simulink model "v3_sim_pi"  (R2023b)
settings: Solver=VariableStepAuto  StartTime=0.0  StopTime=100  RelTol=1e-3
libraries: simulink x1
settings Model: Creator=kiraa  LastModifiedBy=kiraa

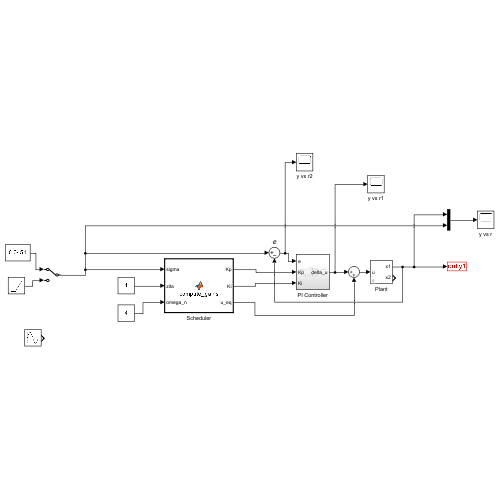
[thumbnail: Simulink's stored preview of the top-level diagram]
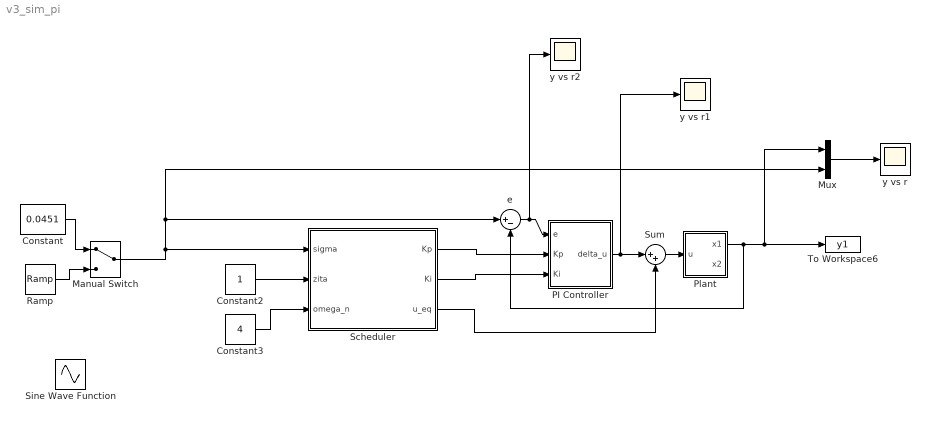
== system v3_sim_pi ==
  Constant : Constant  Value=0.0451
  Constant2 : Constant
  Constant3 : Constant  Value=4
  Manual Switch : ManualSwitch
  Mux : Mux  Inputs=2
  PI Controller : Subsystem
  Plant : Subsystem  mask{x1_0=0, x2_0=0}
      mask prompts: x1_0 "x1(0) [g/l]"; x2_0 "x2(0) [min^-1]"
  Ramp : simulink/Sources/Ramp  slope=0.00001  start=0  InitialOutput=0
  Scheduler : MATLAB Function  TreatAsAtomicUnit=on
  Sine Wave Function : Sin  Amplitude=0.001  Bias=0.0451  Frequency=0.1  SampleTime=0
  Sum : Sum  Inputs=|++
  To Workspace6 : ToWorkspace  VariableName=y1  SaveFormat=Timeseries  SampleTime=-1
  e : Sum  Inputs=|+-
  y vs r : Scope
  y vs r1 : Scope
  y vs r2 : Scope
  wires:
  Plant/1(x1) -> Mux/1, To Workspace6/1, e/2
  Mux/1 -> y vs r/1
  Constant/1 -> Manual Switch/1
  Manual Switch/1 -> Mux/2, e/1, Scheduler/1(sigma)
  Scheduler/1(Kp) -> PI Controller/2(Kp)
  Scheduler/2(Ki) -> PI Controller/3(Ki)
  Constant2/1 -> Scheduler/2(zita)
  Constant3/1 -> Scheduler/3(omega_n)
  Scheduler/3(u_eq) -> Sum/2
  PI Controller/1(delta_u) -> Sum/1, y vs r1/1
  e/1 -> y vs r2/1, PI Controller/1(e)
  Ramp/1 -> Manual Switch/2
  Sum/1 -> Plant/1(u)

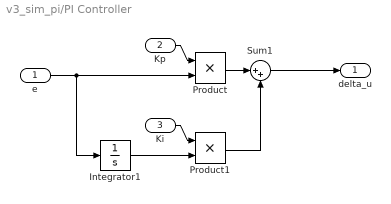
== system v3_sim_pi/PI Controller ==
  e : Inport
  Kp : Inport  Port=2
  Ki : Inport  Port=3
  Integrator1 : Integrator
  Product : Product
  Product1 : Product
  Sum1 : Sum  Inputs=|++
  delta_u : Outport
  wires:
  Product1/1 -> Sum1/2
  e/1 -> Product/2, Integrator1/1
  Integrator1/1 -> Product1/2
  Product/1 -> Sum1/1
  Ki/1 -> Product1/1
  Sum1/1 -> delta_u/1
  Kp/1 -> Product/1

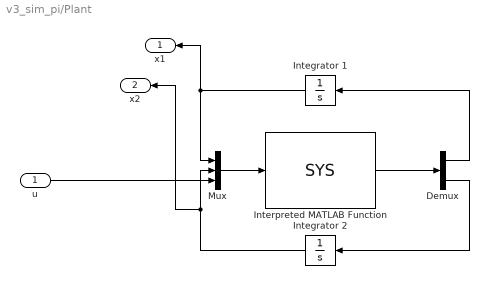
== system v3_sim_pi/Plant ==
  u : Inport
  Demux : Demux  Outputs=2
  Integrator 1 : Integrator  InitialCondition=x1_0
  Integrator 2 : Integrator  InitialCondition=x2_0
  Interpreted MATLAB Function : MATLABFcn  MATLABFcn=SYS  OutputDimensions=2
  Mux : Mux  Inputs=3
  x1 : Outport
  x2 : Outport  Port=2
  wires:
  Integrator 1/1 -> x1/1, Mux/1
  Demux/1 -> Integrator 1/1
  Mux/1 -> Interpreted MATLAB Function/1
  Integrator 2/1 -> x2/1, Mux/2
  Interpreted MATLAB Function/1 -> Demux/1
  Demux/2 -> Integrator 2/1
  u/1 -> Mux/3

== matlab function v3_sim_pi/Scheduler ==
  data: sigma input; Kp output; zita input; omega_n input; Ki output; u_eq output
function [Kp,Ki,u_eq] = compute_gains(sigma, zita, omega_n)
    Kp=-100;
    Ki=0.001;
    u_eq = -(399496308545527218176*sigma - 412936040625518808125)/(8736983277098762240000*sigma);
end
